simulink model "Proyecto_R2018a"  (R2018a)
settings: Solver=VariableStepAuto  StartTime=0.0  StopTime=3
undefined symbols (not defined in the file): alfa_inicial, area_mem, c, cte_kp, d, delta_f, fs, k, m, perm, Q, r1, r_ambiente1, r_ambiente2, rho, v_sonido, vel_caminata, ventana_fft, ventana_fft_analisis, zoh_freq
libraries: dspvision x10, dspmtrx3 x4, dspxfrm3 x3
settings Model: PacingRate=0.110000  Creator=tobip  LastModifiedBy=tobip
settings SolverCC: SolverResetMethod=Robust
settings DataIOCC: ReturnWorkspaceOutputs=on
settings DebuggingCC: UnconnectedInputMsg=none  UnconnectedOutputMsg=none  UnconnectedLineMsg=none
settings ModelReferenceCC: EnableRefExpFcnMdlSchedulingChecks=off
settings SFSimCC: SimUseLocalCustomCode=on
settings RTWCC: Description=Generic Real-Time Target  RTWUseLocalCustomCode=on

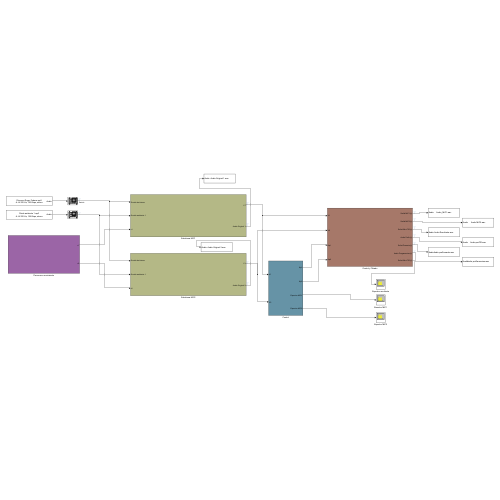
[thumbnail: Simulink's stored preview of the top-level diagram]
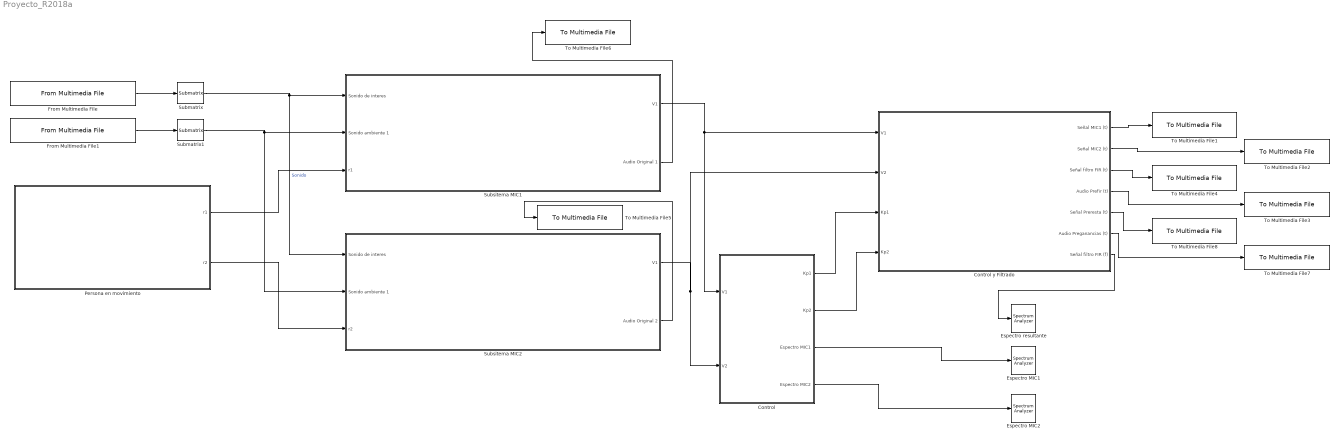
== system Proyecto_R2018a ==
  Control : Subsystem
  Control y Filtrado : Subsystem
  Espectro MIC1 : SpectrumAnalyzer  DefaultConfigurationName=spbscopes.SpectrumAnalyzerBlockCfg
  Espectro MIC2 : SpectrumAnalyzer  DefaultConfigurationName=spbscopes.SpectrumAnalyzerBlockCfg
  Espectro resultante : SpectrumAnalyzer  DefaultConfigurationName=spbscopes.SpectrumAnalyzerBlockCfg
  From Multimedia File : dspvision/From Multimedia File  inputFilename=C:\Users\tobip\Documents\Control\Proyecto final\Audios dato\Discurso Roger Federer.mp3  loop=on  numPlays=1  outputStreams=Audio only  videoDataType=single  audioDataType=double  inheritSampleTime=on  userDefinedSampleTime=1/30  noAudioOutput=off  isIntensityVideo=off  fourcc=RGB  colorVideoFormat=Separate color signals  outputEOF=off  dataOrg=Column-major  audioFrameSize=1  computeAudioFrameSize=off  outSamplingMode=Sample based
  From Multimedia File1 : dspvision/From Multimedia File  inputFilename=C:\Users\tobip\Documents\Control\Proyecto final\Audios dato\Ruido ambiente 1.mp3  loop=on  numPlays=1  outputStreams=Audio only  videoDataType=single  audioDataType=double  inheritSampleTime=on  userDefinedSampleTime=1/30  noAudioOutput=off  isIntensityVideo=off  fourcc=RGB  colorVideoFormat=Separate color signals  outputEOF=off  dataOrg=Column-major  audioFrameSize=1  computeAudioFrameSize=off  outSamplingMode=Sample based
  Persona en movimiento : Subsystem
  Submatrix : dspmtrx3/Submatrix  RowSpan=All rows  RowStartMode=First  RowStartIndex=1  RowEndMode=Middle  RowEndIndex=1  ColSpan=One column  ColStartMode=First  ColStartIndex=1  ColEndMode=Last  ColEndIndex=1
  Submatrix1 : dspmtrx3/Submatrix  RowSpan=All rows  RowStartMode=First  RowStartIndex=1  RowEndMode=Last  RowEndIndex=1  ColSpan=One column  ColStartMode=First  ColStartIndex=1  ColEndMode=Last  ColEndIndex=1
  Subsitema MIC1 : Subsystem
  Subsitema MIC2 : Subsystem
  To Multimedia File1 : dspvision/To Multimedia File  outputFilename=C:\Users\tobip\Documents\Control\Proyecto final\Audio_MIC1.wav  streamSelection=Audio only  videoCompressor=None (uncompressed)  audioCompressor=None (uncompressed)  imagePorts=Separate color signals  fileType=WAV  audioDatatype=16-bit integer  fourcc=RGB  videoQuality=75  mj2000CompFactor=10
  To Multimedia File2 : dspvision/To Multimedia File  outputFilename=C:\Users\tobip\Documents\Control\Proyecto final\Audio MIC2.wav  streamSelection=Audio only  videoCompressor=None (uncompressed)  audioCompressor=None (uncompressed)  imagePorts=Separate color signals  fileType=WAV  audioDatatype=16-bit integer  fourcc=RGB  videoQuality=75  mj2000CompFactor=10
  To Multimedia File3 : dspvision/To Multimedia File  outputFilename=C:\Users\tobip\Documents\Control\Proyecto final\Audio preFIR.wav  streamSelection=Audio only  videoCompressor=None (uncompressed)  audioCompressor=None (uncompressed)  imagePorts=Separate color signals  fileType=WAV  audioDatatype=16-bit integer  fourcc=RGB  videoQuality=75  mj2000CompFactor=10
  To Multimedia File4 : dspvision/To Multimedia File  outputFilename=C:\Users\tobip\Documents\Control\Proyecto final\Audio Resultante.wav  streamSelection=Audio only  videoCompressor=None (uncompressed)  audioCompressor=None (uncompressed)  imagePorts=Separate color signals  fileType=WAV  audioDatatype=16-bit integer  fourcc=RGB  videoQuality=75  mj2000CompFactor=10
  To Multimedia File5 : dspvision/To Multimedia File  outputFilename=C:\Users\tobip\Documents\Control\Proyecto final\Audio Original 2.wav  streamSelection=Audio only  videoCompressor=None (uncompressed)  audioCompressor=None (uncompressed)  imagePorts=Separate color signals  fileType=WAV  audioDatatype=16-bit integer  fourcc=RGB  videoQuality=75  mj2000CompFactor=10
  To Multimedia File6 : dspvision/To Multimedia File  outputFilename=C:\Users\tobip\Documents\Control\Proyecto final\Audio Original 1.wav  streamSelection=Audio only  videoCompressor=None (uncompressed)  audioCompressor=None (uncompressed)  imagePorts=Separate color signals  fileType=WAV  audioDatatype=16-bit integer  fourcc=RGB  videoQuality=75  mj2000CompFactor=10
  To Multimedia File7 : dspvision/To Multimedia File  outputFilename=C:\Users\tobip\Documents\Control\Proyecto final\Audio preGanancias.wav  streamSelection=Audio only  videoCompressor=None (uncompressed)  audioCompressor=None (uncompressed)  imagePorts=Separate color signals  fileType=WAV  audioDatatype=16-bit integer  fourcc=RGB  videoQuality=75  mj2000CompFactor=10
  To Multimedia File8 : dspvision/To Multimedia File  outputFilename=C:\Users\tobip\Documents\Control\Proyecto final\Audio preSumador.wav  streamSelection=Audio only  videoCompressor=None (uncompressed)  audioCompressor=None (uncompressed)  imagePorts=Separate color signals  fileType=WAV  audioDatatype=16-bit integer  fourcc=RGB  videoQuality=75  mj2000CompFactor=10
  wires:
  From Multimedia File/1 -> Submatrix/1
  From Multimedia File1/1 -> Submatrix1/1
  Submatrix/1 -> Subsitema MIC1/1(Sonido de interes), Subsitema MIC2/1(Sonido de interes)  "Sonido"
  Persona en movimiento/1(r1) -> Subsitema MIC1/3(r1)
  Control y Filtrado/1(Señal MIC1 (t)) -> To Multimedia File1/1
  Control y Filtrado/2(Señal MIC2 (t)) -> To Multimedia File2/1
  Control y Filtrado/3(Señal filtro FIR (t)) -> To Multimedia File4/1
  Control y Filtrado/4(Audio Prefir (t)) -> To Multimedia File3/1
  Control y Filtrado/7(Señal filtro FIR (f)) -> Espectro resultante/1
  Submatrix1/1 -> Subsitema MIC1/2(Sonido ambiente 1), Subsitema MIC2/2(Sonido ambiente 1)
  Persona en movimiento/2(r2) -> Subsitema MIC2/3(r2)
  Subsitema MIC1/2(Audio Original 1) -> To Multimedia File6/1
  Subsitema MIC2/2(Audio Original 2) -> To Multimedia File5/1
  Subsitema MIC1/1(V1) -> Control y Filtrado/1(V1), Control/1(V1)
  Subsitema MIC2/1(V1) -> Control y Filtrado/2(V2), Control/2(V2)
  Control/1(Kp1) -> Control y Filtrado/3(Kp1)
  Control/2(Kp2) -> Control y Filtrado/4(Kp2)
  Control/3(Espectro MIC1) -> Espectro MIC1/1
  Control/4(Espectro MIC2) -> Espectro MIC2/1
  Control y Filtrado/5(Señal Preresta (t)) -> To Multimedia File8/1
  Control y Filtrado/6(Audio Preganancias (t)) -> To Multimedia File7/1

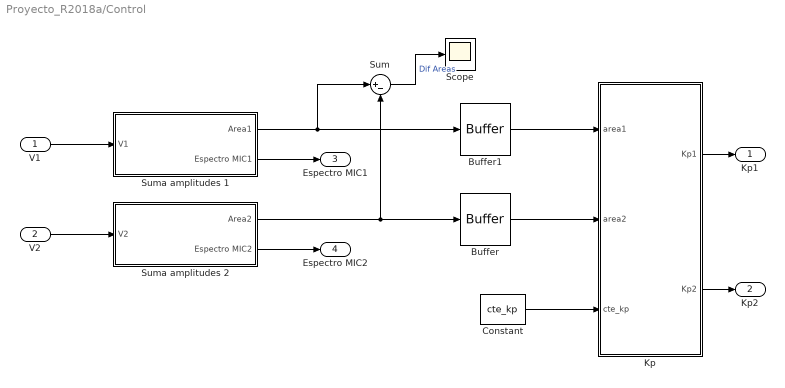
== system Proyecto_R2018a/Control ==
  V1 : Inport
  V2 : Inport  Port=2
  Buffer : Buffer  N=10  V=9  OutputFrames=off
  Buffer1 : Buffer  N=10  V=9  OutputFrames=off
  Constant : Constant  Value=cte_kp
  Kp : MATLAB Function  TreatAsAtomicUnit=on
  Scope : Scope
  Sum : Sum  Inputs=|+-
  Suma amplitudes 1 : Subsystem
  Suma amplitudes 2 : Subsystem
  Kp1 : Outport
  Kp2 : Outport  Port=2
  Espectro MIC1 : Outport  Port=3
  Espectro MIC2 : Outport  Port=4
  wires:
  Kp/1(Kp1) -> Kp1/1
  Constant/1 -> Kp/3(cte_kp)
  V1/1 -> Suma amplitudes 1/1(V1)
  V2/1 -> Suma amplitudes 2/1(V2)
  Kp/2(Kp2) -> Kp2/1
  Suma amplitudes 1/2(Espectro MIC1) -> Espectro MIC1/1
  Suma amplitudes 2/2(Espectro MIC2) -> Espectro MIC2/1
  Sum/1 -> Scope/1  "Dif Areas"
  Suma amplitudes 1/1(Area1) -> Buffer1/1, Sum/1
  Suma amplitudes 2/1(Area2) -> Sum/2, Buffer/1
  Buffer/1 -> Kp/2(area2)
  Buffer1/1 -> Kp/1(area1)

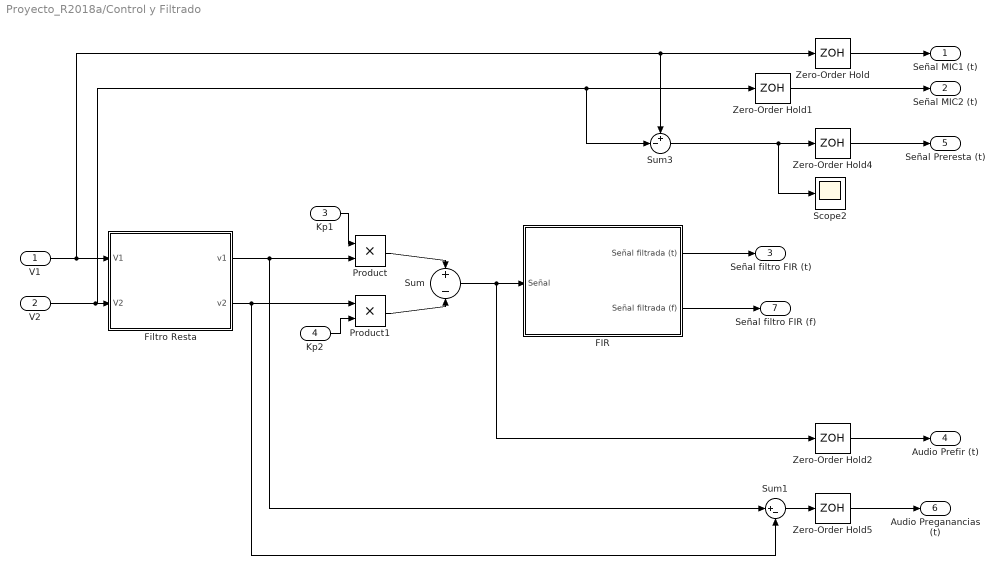
== system Proyecto_R2018a/Control y Filtrado ==
  V1 : Inport
  V2 : Inport  Port=2
  Kp1 : Inport  Port=3
  Kp2 : Inport  Port=4
  FIR : Subsystem
  Filtro Resta : MATLAB Function  TreatAsAtomicUnit=on
  Product : Product
  Product1 : Product
  Scope2 : Scope
  Sum : Sum  Inputs=+-
  Sum1 : Sum  Inputs=|+-
  Sum3 : Sum  Inputs=+-|
  Zero-Order Hold{,1..2,5} (4 alike) : ZeroOrderHold  SampleTime=1/fs
  Zero-Order Hold4 : ZeroOrderHold  SampleTime=1/44100
  Señal MIC1 (t) : Outport
  Señal MIC2 (t) : Outport  Port=2
  Señal filtro FIR (t) : Outport  Port=3
  Audio Prefir (t) : Outport  Port=4
  Señal Preresta (t) : Outport  Port=5
  Audio Preganancias (t) : Outport  Port=6
  Señal filtro FIR (f) : Outport  Port=7
  wires:
  V2/1 -> Filtro Resta/2(V2), Sum3/2, Zero-Order Hold1/1
  V1/1 -> Sum3/1, Zero-Order Hold/1, Filtro Resta/1(V1)
  Sum/1 -> FIR/1(Señal), Zero-Order Hold2/1
  FIR/2(Señal filtrada (f)) -> Señal filtro FIR (f)/1
  FIR/1(Señal filtrada (t)) -> Señal filtro FIR (t)/1
  Filtro Resta/2(v2) -> Product1/1, Sum1/2
  Filtro Resta/1(v1) -> Product/2, Sum1/1
  Zero-Order Hold/1 -> Señal MIC1 (t)/1
  Zero-Order Hold1/1 -> Señal MIC2 (t)/1
  Zero-Order Hold2/1 -> Audio Prefir (t)/1
  Sum1/1 -> Zero-Order Hold5/1
  Product1/1 -> Sum/2
  Product/1 -> Sum/1
  Sum3/1 -> Zero-Order Hold4/1, Scope2/1
  Kp1/1 -> Product/1
  Kp2/1 -> Product1/2
  Zero-Order Hold4/1 -> Señal Preresta (t)/1
  Zero-Order Hold5/1 -> Audio Preganancias (t)/1

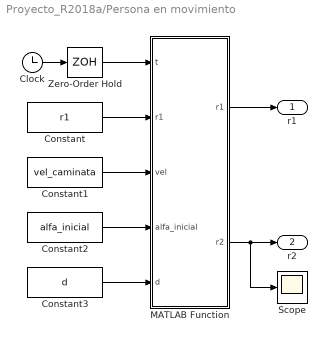
== system Proyecto_R2018a/Persona en movimiento ==
  Clock : Clock
  Constant : Constant  Value=r1
  Constant1 : Constant  Value=vel_caminata
  Constant2 : Constant  Value=alfa_inicial
  Constant3 : Constant  Value=d
  MATLAB Function : MATLAB Function  TreatAsAtomicUnit=on
  Scope : Scope
  Zero-Order Hold : ZeroOrderHold  SampleTime=0.1
  r1 : Outport
  r2 : Outport  Port=2
  wires:
  Constant/1 -> MATLAB Function/2("r1 ")
  Constant3/1 -> MATLAB Function/5(d)
  Constant2/1 -> MATLAB Function/4(alfa_inicial)
  Constant1/1 -> MATLAB Function/3(vel)
  Clock/1 -> Zero-Order Hold/1
  MATLAB Function/1(r1) -> r1/1
  Zero-Order Hold/1 -> MATLAB Function/1(t)
  MATLAB Function/2(r2) -> r2/1, Scope/1

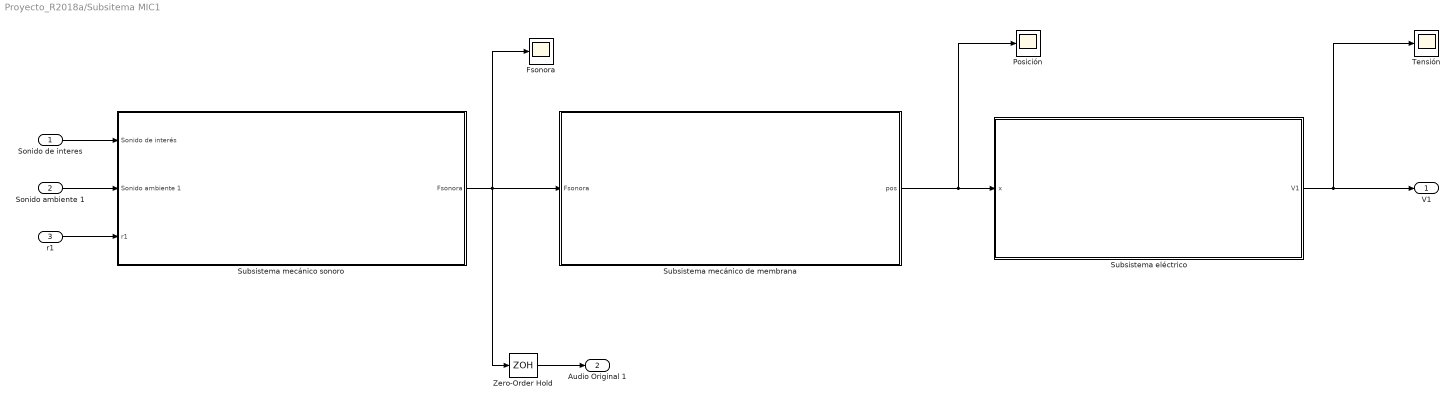
== system Proyecto_R2018a/Subsitema MIC1 ==
  Sonido de interes : Inport
  Sonido ambiente 1 : Inport  Port=2
  r1 : Inport  Port=3
  Fsonora : Scope
  Posición : Scope
  Subsistema eléctrico : Subsystem
  Subsistema mecánico de membrana : Subsystem
  Subsistema mecánico sonoro : Subsystem
  Tensión : Scope
  Zero-Order Hold : ZeroOrderHold  SampleTime=1/fs
  V1 : Outport
  Audio Original 1 : Outport  Port=2
  wires:
  Subsistema mecánico de membrana/1(pos) -> Posición/1, Subsistema eléctrico/1(x)
  Sonido de interes/1 -> Subsistema mecánico sonoro/1(Sonido de interés)
  Subsistema eléctrico/1(V1) -> Tensión/1, V1/1
  Subsistema mecánico sonoro/1(Fsonora) -> Fsonora/1, Zero-Order Hold/1, Subsistema mecánico de membrana/1(Fsonora)
  Sonido ambiente 1/1 -> Subsistema mecánico sonoro/2(Sonido ambiente 1)
  r1/1 -> Subsistema mecánico sonoro/3(r1)
  Zero-Order Hold/1 -> Audio Original 1/1

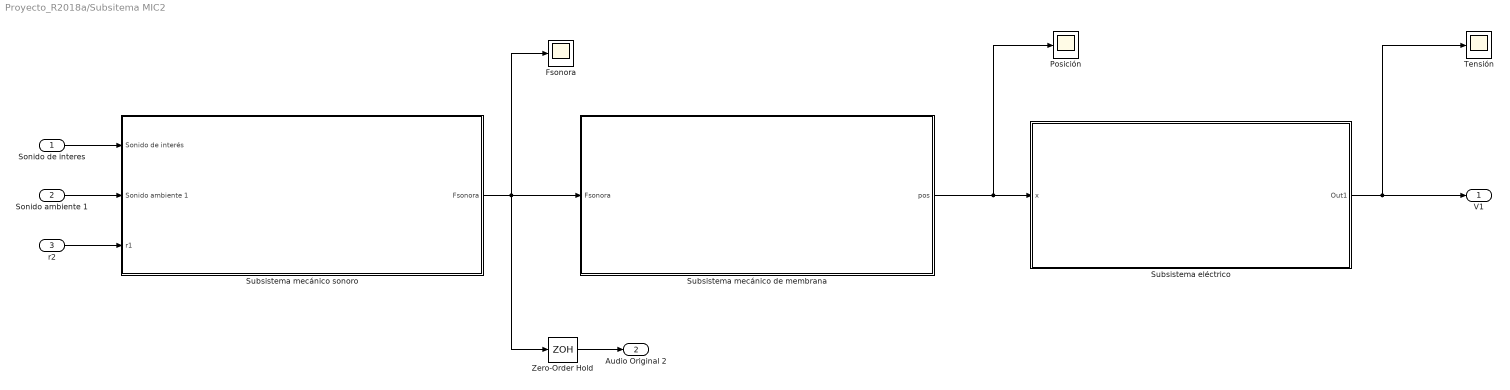
== system Proyecto_R2018a/Subsitema MIC2 ==
  Sonido de interes : Inport
  Sonido ambiente 1 : Inport  Port=2
  r2 : Inport  Port=3
  Fsonora : Scope
  Posición : Scope
  Subsistema eléctrico : Subsystem
  Subsistema mecánico de membrana : Subsystem
  Subsistema mecánico sonoro : Subsystem
  Tensión : Scope
  Zero-Order Hold : ZeroOrderHold  SampleTime=1/fs
  V1 : Outport
  Audio Original 2 : Outport  Port=2
  wires:
  Subsistema mecánico de membrana/1(pos) -> Posición/1, Subsistema eléctrico/1(x)
  Sonido de interes/1 -> Subsistema mecánico sonoro/1(Sonido de interés)
  Subsistema eléctrico/1(Out1) -> Tensión/1, V1/1
  Subsistema mecánico sonoro/1(Fsonora) -> Zero-Order Hold/1, Fsonora/1, Subsistema mecánico de membrana/1(Fsonora)
  Sonido ambiente 1/1 -> Subsistema mecánico sonoro/2(Sonido ambiente 1)
  r2/1 -> Subsistema mecánico sonoro/3(r1)
  Zero-Order Hold/1 -> Audio Original 2/1

== system Proyecto_R2018a/Control/Suma amplitudes 1 ==
  V1 : Inport
  Constant : Constant  Value=delta_f
  FFT : Subsystem
  MATLAB Function : MATLAB Function  TreatAsAtomicUnit=on
  Sum of Elements : Sum  Inputs=+
  Area1 : Outport
  Espectro MIC1 : Outport  Port=2
  wires:
  FFT/1(A) -> MATLAB Function/1(A)
  Constant/1 -> MATLAB Function/2(delta_f)
  MATLAB Function/1(areas) -> Sum of Elements/1
  Sum of Elements/1 -> Area1/1
  V1/1 -> FFT/1(In1)
  FFT/2(MIC1) -> Espectro MIC1/1

== system Proyecto_R2018a/Control/Suma amplitudes 2 ==
  V2 : Inport
  Constant : Constant  Value=delta_f
  MATLAB Function : MATLAB Function  TreatAsAtomicUnit=on
  Subsystem : Subsystem
  Sum of Elements : Sum  Inputs=+
  Area2 : Outport
  Espectro MIC2 : Outport  Port=2
  wires:
  Subsystem/1(A) -> MATLAB Function/1(A)
  Constant/1 -> MATLAB Function/2(delta_f)
  MATLAB Function/1(areas) -> Sum of Elements/1
  Sum of Elements/1 -> Area2/1
  V2/1 -> Subsystem/1(In1)
  Subsystem/2(MIC2) -> Espectro MIC2/1

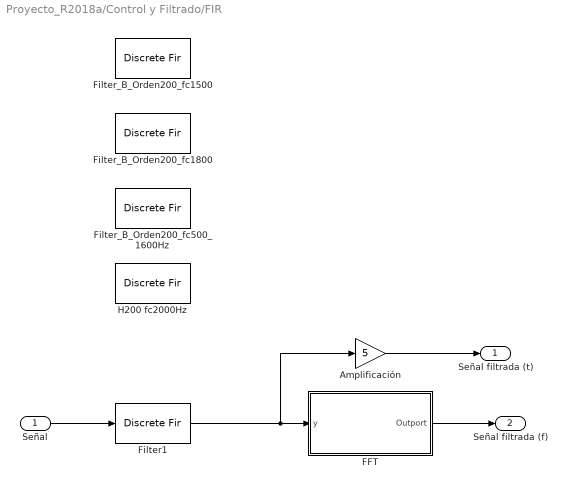
== system Proyecto_R2018a/Control y Filtrado/FIR ==
  Señal : Inport
  Amplificación : Gain  Gain=5
  FFT : Subsystem
  Filter1 : DiscreteFir  Tag=BlockMethodSubSystem  Coefficients=[0 -2.46968087486229999e-06 -3.07570330301983584e-05 -0.000118398297516965302 -0.000298367075036484037 -0.000596227803309950849 -0.00102003077952711506 -0.00154756625881359144 -0.00211289076768585247 -0.00259518747306043901 -0.00281365562212182018 -0.00253195194747434741 -0.00147460264563965674 0.00064414461322387991 0.00408104805501018075 0.00901875177176652762 0.0155214581908035953 0.0234991010213631106 0.0326874432853242192 0.0426497872392069197 0.0528029801451961808 0.0624665952648715134 0.070930220073032374 0.0775304241645051739 0.0817268652809263335 0.0831665725577227094 0.0817268652809263335 0.0775304241645051739 0.070930220073032374 0.0624665952648715134 0.0528029801451961808 0.0426497872392069197 0.0326874432853242192 0.0234991010213631106 0.0155214581908035953 0.00901875177176652762 0.00408104805501018075 0.00064414461322387991 -0.00147460264563965674 -0.00253195194747434741 -0.00281365562212182018 -0.00259518747306043901 -0.00211289076768585247 -0.00154756625881359144 -0.00102003077952711506 -0.000596227803309950849 -0.000298367075036484037 -0.000118398297516965302 -3.07570330301983584e-05 -2.46968087486229999e-06 0]
  Filter_B_Orden200_fc1500 : DiscreteFir  Tag=BlockMethodSubSystem  Coefficients=[0 2.11514125222930549e-07 1.00093934765138096e-06 2.50662436979156886e-06 4.71763254290821587e-06 7.45535130819729324e-06 1.03710140877794857e-05 1.2960590087806268e-05 1.45973519410186672e-05 1.45811762675124996e-05 1.22023273134778345e-05 6.81618827244323951e-06 -2.07578339154207704e-06 -1.47446077930910027e-05 -3.11583144423782112e-05 -5.09193211148811369e-05 -7.32215020803920553e-05 -9.68332887952996719e-05 -0.000120112140303127817 -0.000141054205202763115 -0.000157381003729514476 -0.000166662556647139825 -0.000166473685437744368 -0.00015457735079446705 -0.000129126060727848284 -8.88697665733315106e-05 -3.33564884044779432e-05 3.68896166032006936e-05 0.000120228712346331866 0.000213819912830098396 0.000313604278663653989 0.000414367756397579403 0.000509891865637218319 0.000593195126311718709 0.000656862556488219465 0.000693454334739479331 0.000695978258336398588 0.000658404344862743309 0.000576194261678405215 0.000446813676266662413 0.000270192532359212259 4.90970521410024542e-05 -0.000210621758123884174 -0.000499934975730347594 -0.000806724111547534105 -0.00111606896143020282 -0.00141074282481386303 -0.00167191115831235291 -0.00188001685492420584 -0.00201582207294112928 -0.00206156366447221876 -0.00200216760345560841 -0.00182645822084354721 -0.0015282913035907222 -0.00110753688360242983 -0.000570838357529814943 6.79202371766113587e-05 0.00078749732174142491 0.00155957185340557065 0.00234944320823486348 0.00311715878165994996 0.00381905210809447421 0.00440965014053728861 0.00484388441406833313 0.00507951851693627058 0.00507968498761981503 0.0048154097481520608 0.00426799261879337762 0.00343110924951585535 0.00231250356255708039 0.000935150787564285099 -0.000662210741248886155 -0.00242525619795645655 -0.00428500615435206331 -0.00615952594606015199 -0.00795636728195464604 -0.00957568849089815606 -0.0109139524588171416 -0.0118680670103581479 -0.0123398031736713185 -0.0122403041952631221 -0.0114944838213977812 -0.0100451073342442999 -0.0078563537756842685 -0.00491667285846230425 -0.00124077487520772665 0.00312937443093690539 0.0081246409678302229 0.0136499315738288548 0.019586515496723484 0.0257953968596963713 0.0321216271410308465 0.0383994009130048802 0.0444577386408763556 0.0501265293153456901 0.0552426847697761667 0.0596561479180048454 0.0632354994835633705 0.065872922121823177 0.067488306600615014 0.0680323207557864684 0.067488306600615014 0.065872922121823177 0.0632354994835633705 0.0596561479180048454 0.0552426847697761667 0.0501265293153456901 0.0444577386408763556 0.0383994009130048802 0.0321216271410308465 0.0257953968596963713 0.019586515496723484 0.0136499315738288548 0.0081246409678302229 0.00312937443093690539 -0.00124077487520772665 -0.00491667285846230425 -0.0078563537756842685 -0.0100451073342442999 -0.0114944838213977812 -0.0122403041952631221 -0.0123398031736713185 -0.0118680670103581479 -0.0109139524588171416 -0.00957568849089815606 -0.00795636728195464604 -0.00615952594606015199 -0.00428500615435206331 -0.00242525619795645655 -0.000662210741248886155 0.000935150787564285099 0.00231250356255708039 0.00343110924951585535 0.00426799261879337762 0.0048154097481520608 0.00507968498761981503 0.00507951851693627058 0.00484388441406833313 0.00440965014053728861 0.00381905210809447421 0.00311715878165994996 0.00234944320823486348 0.00155957185340557065 0.00078749732174142491 6.79202371766113587e-05 -0.000570838357529814943 -0.00110753688360242983 -0.0015282913035907222 -0.00182645822084354721 -0.00200216760345560841 -0.00206156366447221876 -0.00201582207294112928 -0.00188001685492420584 -0.00167191115831235291 -0.00141074282481386303 -0.00111606896143020282 -0.000806724111547534105 -0.000499934975730347594 -0.000210621758123884174 4.90970521410024542e-05 0.000270192532359212259 0.000446813676266662413 0.000576194261678405215 0.000658404344862743309 0.000695978258336398588 0.000693454334739479331 0.000656862556488219465 0.000593195126311718709 0.000509891865637218319 0.000414367756397579403 0.000313604278663653989 ...(+711 chars)]
  Filter_B_Orden200_fc1800 : DiscreteFir  Tag=BlockMethodSubSystem  Coefficients=[0 2.11514125222930549e-07 1.00093934765138096e-06 2.50662436979156886e-06 4.71763254290821587e-06 7.45535130819729324e-06 1.03710140877794857e-05 1.2960590087806268e-05 1.45973519410186672e-05 1.45811762675124996e-05 1.22023273134778345e-05 6.81618827244323951e-06 -2.07578339154207704e-06 -1.47446077930910027e-05 -3.11583144423782112e-05 -5.09193211148811369e-05 -7.32215020803920553e-05 -9.68332887952996719e-05 -0.000120112140303127817 -0.000141054205202763115 -0.000157381003729514476 -0.000166662556647139825 -0.000166473685437744368 -0.00015457735079446705 -0.000129126060727848284 -8.88697665733315106e-05 -3.33564884044779432e-05 3.68896166032006936e-05 0.000120228712346331866 0.000213819912830098396 0.000313604278663653989 0.000414367756397579403 0.000509891865637218319 0.000593195126311718709 0.000656862556488219465 0.000693454334739479331 0.000695978258336398588 0.000658404344862743309 0.000576194261678405215 0.000446813676266662413 0.000270192532359212259 4.90970521410024542e-05 -0.000210621758123884174 -0.000499934975730347594 -0.000806724111547534105 -0.00111606896143020282 -0.00141074282481386303 -0.00167191115831235291 -0.00188001685492420584 -0.00201582207294112928 -0.00206156366447221876 -0.00200216760345560841 -0.00182645822084354721 -0.0015282913035907222 -0.00110753688360242983 -0.000570838357529814943 6.79202371766113587e-05 0.00078749732174142491 0.00155957185340557065 0.00234944320823486348 0.00311715878165994996 0.00381905210809447421 0.00440965014053728861 0.00484388441406833313 0.00507951851693627058 0.00507968498761981503 0.0048154097481520608 0.00426799261879337762 0.00343110924951585535 0.00231250356255708039 0.000935150787564285099 -0.000662210741248886155 -0.00242525619795645655 -0.00428500615435206331 -0.00615952594606015199 -0.00795636728195464604 -0.00957568849089815606 -0.0109139524588171416 -0.0118680670103581479 -0.0123398031736713185 -0.0122403041952631221 -0.0114944838213977812 -0.0100451073342442999 -0.0078563537756842685 -0.00491667285846230425 -0.00124077487520772665 0.00312937443093690539 0.0081246409678302229 0.0136499315738288548 0.019586515496723484 0.0257953968596963713 0.0321216271410308465 0.0383994009130048802 0.0444577386408763556 0.0501265293153456901 0.0552426847697761667 0.0596561479180048454 0.0632354994835633705 0.065872922121823177 0.067488306600615014 0.0680323207557864684 0.067488306600615014 0.065872922121823177 0.0632354994835633705 0.0596561479180048454 0.0552426847697761667 0.0501265293153456901 0.0444577386408763556 0.0383994009130048802 0.0321216271410308465 0.0257953968596963713 0.019586515496723484 0.0136499315738288548 0.0081246409678302229 0.00312937443093690539 -0.00124077487520772665 -0.00491667285846230425 -0.0078563537756842685 -0.0100451073342442999 -0.0114944838213977812 -0.0122403041952631221 -0.0123398031736713185 -0.0118680670103581479 -0.0109139524588171416 -0.00957568849089815606 -0.00795636728195464604 -0.00615952594606015199 -0.00428500615435206331 -0.00242525619795645655 -0.000662210741248886155 0.000935150787564285099 0.00231250356255708039 0.00343110924951585535 0.00426799261879337762 0.0048154097481520608 0.00507968498761981503 0.00507951851693627058 0.00484388441406833313 0.00440965014053728861 0.00381905210809447421 0.00311715878165994996 0.00234944320823486348 0.00155957185340557065 0.00078749732174142491 6.79202371766113587e-05 -0.000570838357529814943 -0.00110753688360242983 -0.0015282913035907222 -0.00182645822084354721 -0.00200216760345560841 -0.00206156366447221876 -0.00201582207294112928 -0.00188001685492420584 -0.00167191115831235291 -0.00141074282481386303 -0.00111606896143020282 -0.000806724111547534105 -0.000499934975730347594 -0.000210621758123884174 4.90970521410024542e-05 0.000270192532359212259 0.000446813676266662413 0.000576194261678405215 0.000658404344862743309 0.000695978258336398588 0.000693454334739479331 0.000656862556488219465 0.000593195126311718709 0.000509891865637218319 0.000414367756397579403 0.000313604278663653989 ...(+711 chars)]
  Filter_B_Orden200_fc500_1600Hz : DiscreteFir  Tag=BlockMethodSubSystem  Coefficients=[0 -3.55324752461809841e-07 -1.14041164662054229e-06 -1.86555151808696453e-06 -1.99844780883798536e-06 -1.03117503681064552e-06 1.45062710751347741e-06 5.70289528973608542e-06 1.17693159029814948e-05 1.94448656927964283e-05 2.82621895124256615e-05 3.75049240470417836e-05 4.62502611344708104e-05 5.34408510414543662e-05 5.79836863954314837e-05 5.88710269009623936e-05 5.53158980566520483e-05 4.68924195295184699e-05 3.36693962809190553e-05 1.63244395128763006e-05 -3.77444374118628878e-06 -2.453220038109486e-05 -4.31457047987660692e-05 -5.61862277492814434e-05 -5.97494327243870303e-05 -4.96722181784016028e-05 -2.18103772002809209e-05 2.76346086120937394e-05 0.000101756893313425151 0.000202578002872316965 0.000330695331954048983 0.000484976370934371733 0.000662328426985930993 0.000857572264827437562 0.00106344444062398498 0.00127074710823718118 0.0014686558861857909 0.00164518631562104219 0.00178780802395475213 0.0018841836077030836 0.0019229972643288473 0.00189482722409228983 0.00179300697511287107 0.00161441401740641485 0.0013601221987472544 0.00103585517795217862 0.000652184596068289225 0.000224427194425909913 -0.00022778983727046132 -0.000681307141145609443 -0.00111054518170260381 -0.00148891652354738281 -0.00179048116367318505 -0.00199176515444643909 -0.00207364314459349474 -0.0020231703767315209 -0.00183524054863001091 -0.00151394393656255908 -0.00107350608403622406 -0.000538701511402984025 5.53408815078556784e-05 0.000663994493666133687 0.00123467192903057438 0.00170902033542422215 0.00202571129447411602 0.00212371962214221886 0.00194594664007262993 0.00144301027073342526 0.000576999157387270015 -0.000675026961659274034 -0.00231801155623287836 -0.00433656156585883468 -0.00669348216553504807 -0.00932933927728997296 -0.0121631565101997467 -0.0150942974724516503 -0.0180055222248230451 -0.0207671413150356775 -0.0232421259844599291 -0.0252919725618051955 -0.0267830664686852619 -0.0275932500724108756 -0.027618271722570361 -0.0267777828722388159 -0.0250205575078153546 -0.0223286335031159487 -0.0187201182440967645 -0.014250459181509658 -0.00901205114390197723 -0.00313213274256277877 0.00323099015437159709 0.00989326969472957042 0.0166515838433948446 0.0232914672367314154 0.0295955653449251239 0.0353524284672399047 0.0403652375807131078 0.04446005042715033 0.0474931739498184249 0.0493573075805954289 0.0499861590665064068 0.0493573075805954289 0.0474931739498184249 0.04446005042715033 0.0403652375807131078 0.0353524284672399047 0.0295955653449251239 0.0232914672367314154 0.0166515838433948446 0.00989326969472957042 0.00323099015437159709 -0.00313213274256277877 -0.00901205114390197723 -0.014250459181509658 -0.0187201182440967645 -0.0223286335031159487 -0.0250205575078153546 -0.0267777828722388159 -0.027618271722570361 -0.0275932500724108756 -0.0267830664686852619 -0.0252919725618051955 -0.0232421259844599291 -0.0207671413150356775 -0.0180055222248230451 -0.0150942974724516503 -0.0121631565101997467 -0.00932933927728997296 -0.00669348216553504807 -0.00433656156585883468 -0.00231801155623287836 -0.000675026961659274034 0.000576999157387270015 0.00144301027073342526 0.00194594664007262993 0.00212371962214221886 0.00202571129447411602 0.00170902033542422215 0.00123467192903057438 0.000663994493666133687 5.53408815078556784e-05 -0.000538701511402984025 -0.00107350608403622406 -0.00151394393656255908 -0.00183524054863001091 -0.0020231703767315209 -0.00207364314459349474 -0.00199176515444643909 -0.00179048116367318505 -0.00148891652354738281 -0.00111054518170260381 -0.000681307141145609443 -0.00022778983727046132 0.000224427194425909913 0.000652184596068289225 0.00103585517795217862 0.0013601221987472544 0.00161441401740641485 0.00179300697511287107 0.00189482722409228983 0.0019229972643288473 0.0018841836077030836 0.00178780802395475213 0.00164518631562104219 0.0014686558861857909 0.00127074710823718118 0.00106344444062398498 0.000857572264827437562 0.000662328426985930993 0.000484976370934371733 0.000330695331954048983 ...(+708 chars)]
  H200 fc2000Hz : DiscreteFir  Tag=BlockMethodSubSystem  Coefficients=[-5.56928887965323996e-05 1.65011438245537004e-05 8.97404129389855278e-05 0.000159235323802665862 0.00022009162972417537 0.000267507778546905491 0.000297028076662561244 0.00030485366062257119 0.000288200030555739591 0.000245675511305965986 0.000177641669329940406 8.6506699720296273e-05 -2.31018469780051173e-05 -0.00014433637834937926 -0.000268342086729793134 -0.000384707364236210015 -0.00048215215755155206 -0.000549426670478966937 -0.000576363543252263362 -0.000554999408859523633 -0.000480660081578202522 -0.000352890851136748013 -0.000176112058154881163 4.01080891230722538e-05 0.0002812463338075579 0.000528528322799664608 0.000760142225443803492 0.000952907949042803453 0.00108429460403765884 0.00113463045342545839 0.00108931159601457291 0.00094079311035012215 0.000690143237104743116 0.000347959694228160642 -6.55123016736293336e-05 -0.000521160190085571311 -0.000982705755809358409 -0.00140926525119598289 -0.00175861601479996091 -0.001990934889977244 -0.00207270564165747606 -0.00198044699745618087 -0.00170389625705465349 -0.00124829972377997456 -0.000635511796707235511 9.63124522686815125e-05 0.000894536087431914602 0.00169534580071897009 0.0024283810074139326 0.00302238837764083959 0.00341148451645994577 0.00354151851327269909 0.00337597368177574393 0.00290084170646281786 0.00212794664955293479 0.00109629064041346963 -0.000128867164522033134 -0.00145931071589772685 -0.00278945929549263881 -0.00400395802404863912 -0.00498677619654774081 -0.00563115432140427145 -0.00584961657959357211 -0.00558319945973669973 -0.00480904907338582793 -0.00354561337216146395 -0.00185479953038198927 0.000159326606607727535 0.00235546635562724864 0.00456352016844470149 0.00659611134894932602 0.00826250699229939302 0.00938400051612865889 0.00980963996366138874 0.00943108496947073389 0.0081953652910344444 0.00611440066924413047 0.00327032343009041803 -0.000184088132840851902 -0.00403022302427255476 -0.00799367568943868192 -0.0117590911319403208 -0.0149890162285861283 -0.0173456171069947714 -0.0185138545635019809 -0.0182245363907261523 -0.0162756038401307805 -0.0125500678039269838 -0.00702918815483403927 0.000200222721545358193 0.0089451122912353586 0.0189124119976689584 0.029721990975099373 0.0409256801261550299 0.052031266702432348 0.0625299886144426165 0.0719257851026266215 0.079764407724826486 0.0856604757140051049 0.0893206756611368557 0.0905615500562179931 0.0893206756611368557 0.0856604757140051049 0.079764407724826486 0.0719257851026266215 0.0625299886144426165 0.052031266702432348 0.0409256801261550299 0.029721990975099373 0.0189124119976689584 0.0089451122912353586 0.000200222721545358193 -0.00702918815483403927 -0.0125500678039269838 -0.0162756038401307805 -0.0182245363907261523 -0.0185138545635019809 -0.0173456171069947714 -0.0149890162285861283 -0.0117590911319403208 -0.00799367568943868192 -0.00403022302427255476 -0.000184088132840851902 0.00327032343009041803 0.00611440066924413047 0.0081953652910344444 0.00943108496947073389 0.00980963996366138874 0.00938400051612865889 0.00826250699229939302 0.00659611134894932602 0.00456352016844470149 0.00235546635562724864 0.000159326606607727535 -0.00185479953038198927 -0.00354561337216146395 -0.00480904907338582793 -0.00558319945973669973 -0.00584961657959357211 -0.00563115432140427145 -0.00498677619654774081 -0.00400395802404863912 -0.00278945929549263881 -0.00145931071589772685 -0.000128867164522033134 0.00109629064041346963 0.00212794664955293479 0.00290084170646281786 0.00337597368177574393 0.00354151851327269909 0.00341148451645994577 0.00302238837764083959 0.0024283810074139326 0.00169534580071897009 0.000894536087431914602 9.63124522686815125e-05 -0.000635511796707235511 -0.00124829972377997456 -0.00170389625705465349 -0.00198044699745618087 -0.00207270564165747606 -0.001990934889977244 -0.00175861601479996091 -0.00140926525119598289 -0.000982705755809358409 -0.000521160190085571311 -6.55123016736293336e-05 0.000347959694228160642 0.000690143237104743116 0.00094079311035012215 ...(+746 chars)]
  Señal filtrada (t) : Outport
  Señal filtrada (f) : Outport  Port=2
  wires:
  FFT/1(Outport) -> Señal filtrada (f)/1
  Amplificación/1 -> Señal filtrada (t)/1
  Señal/1 -> Filter1/1
  Filter1/1 -> Amplificación/1, FFT/1(y)

== system Proyecto_R2018a/Subsitema MIC1/Subsistema eléctrico ==
  x : Inport
  Constant : Constant  Value=area_mem*perm
  Constant1 : Constant  Value=Q
  Divide : Product  Inputs=*/
  Divide1 : Product  Inputs=*/
  V1 : Outport
  wires:
  x/1 -> Divide/2
  Constant/1 -> Divide/1
  Divide/1 -> Divide1/2  "Capacitancia"
  Divide1/1 -> V1/1
  Constant1/1 -> Divide1/1

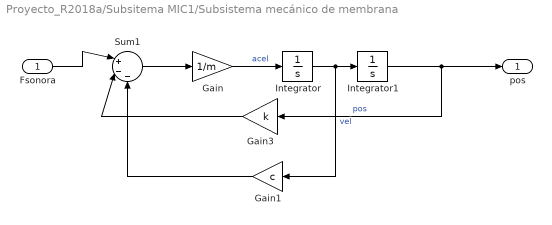
== system Proyecto_R2018a/Subsitema MIC1/Subsistema mecánico de membrana ==
  Fsonora : Inport
  Gain : Gain  Gain=1/m
  Gain1 : Gain  Gain=c
  Gain3 : Gain  Gain=k
  Integrator : Integrator
  Integrator1 : Integrator
  Sum1 : Sum  Inputs=|+--
  pos : Outport
  wires:
  Integrator1/1 -> Gain3/1, pos/1  "pos"
  Integrator/1 -> Gain1/1, Integrator1/1  "vel"
  Fsonora/1 -> Sum1/1
  Gain3/1 -> Sum1/2
  Sum1/1 -> Gain/1
  Gain/1 -> Integrator/1  "acel"
  Gain1/1 -> Sum1/3

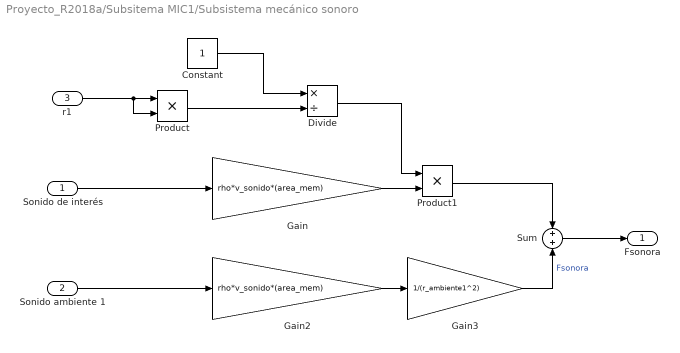
== system Proyecto_R2018a/Subsitema MIC1/Subsistema mecánico sonoro ==
  Sonido de interés : Inport
  Sonido ambiente 1 : Inport  Port=2
  r1 : Inport  Port=3
  Constant : Constant
  Divide : Product  Inputs=*/
  Gain : Gain  Gain=rho*v_sonido*(area_mem)
  Gain2 : Gain  Gain=rho*v_sonido*(area_mem)
  Gain3 : Gain  Gain=1/(r_ambiente1^2)
  Product : Product
  Product1 : Product
  Sum : Sum
  Fsonora : Outport
  wires:
  Gain/1 -> Product1/2
  Sonido de interés/1 -> Gain/1
  Gain2/1 -> Gain3/1
  Gain3/1 -> Sum/2  "Fsonora"
  Sonido ambiente 1/1 -> Gain2/1
  Sum/1 -> Fsonora/1
  r1/1 -> Product/2, Product/1
  Product/1 -> Divide/2
  Constant/1 -> Divide/1
  Divide/1 -> Product1/1
  Product1/1 -> Sum/1

== system Proyecto_R2018a/Subsitema MIC2/Subsistema eléctrico ==
  x : Inport
  Constant : Constant  Value=area_mem*perm
  Constant1 : Constant  Value=Q
  Divide : Product  Inputs=*/
  Divide1 : Product  Inputs=*/
  Out1 : Outport
  wires:
  x/1 -> Divide/2
  Constant/1 -> Divide/1
  Divide/1 -> Divide1/2  "Capacitancia"
  Divide1/1 -> Out1/1
  Constant1/1 -> Divide1/1

== system Proyecto_R2018a/Subsitema MIC2/Subsistema mecánico de membrana ==
  Fsonora : Inport
  Gain : Gain  Gain=1/m
  Gain1 : Gain  Gain=c
  Gain3 : Gain  Gain=k
  Integrator : Integrator
  Integrator1 : Integrator
  Sum1 : Sum  Inputs=|+--
  pos : Outport
  wires:
  Integrator1/1 -> Gain3/1, pos/1  "pos"
  Integrator/1 -> Gain1/1, Integrator1/1  "vel"
  Fsonora/1 -> Sum1/1
  Gain3/1 -> Sum1/2
  Sum1/1 -> Gain/1
  Gain/1 -> Integrator/1  "acel"
  Gain1/1 -> Sum1/3

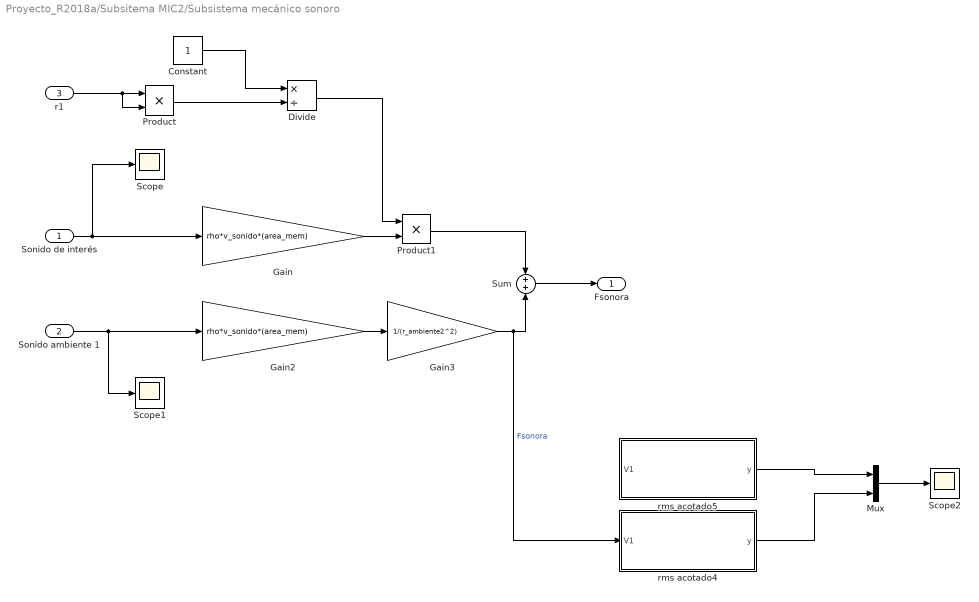
== system Proyecto_R2018a/Subsitema MIC2/Subsistema mecánico sonoro ==
  Sonido de interés : Inport
  Sonido ambiente 1 : Inport  Port=2
  r1 : Inport  Port=3
  Constant : Constant
  Divide : Product  Inputs=*/
  Gain : Gain  Gain=rho*v_sonido*(area_mem)
  Gain2 : Gain  Gain=rho*v_sonido*(area_mem)
  Gain3 : Gain  Gain=1/(r_ambiente2^2)
  Mux : Mux  Inputs=2
  Product : Product
  Product1 : Product
  Scope : Scope
  Scope1 : Scope
  Scope2 : Scope
  Sum : Sum
  rms acotado4 : Subsystem
  rms acotado5 : Subsystem
  Fsonora : Outport
  wires:
  Gain/1 -> Product1/2
  Sonido de interés/1 -> Gain/1, Scope/1
  Gain2/1 -> Gain3/1
  Gain3/1 -> rms acotado4/1(V1), Sum/2  "Fsonora"
  Sonido ambiente 1/1 -> Scope1/1, Gain2/1
  Sum/1 -> Fsonora/1
  rms acotado5/1(y) -> Mux/1
  rms acotado4/1(y) -> Mux/2
  Mux/1 -> Scope2/1
  r1/1 -> Product/2, Product/1
  Product/1 -> Divide/2
  Constant/1 -> Divide/1
  Divide/1 -> Product1/1
  Product1/1 -> Sum/1

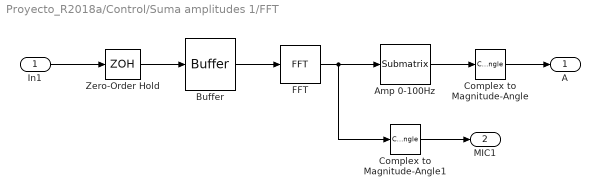
== system Proyecto_R2018a/Control/Suma amplitudes 1/FFT ==
  In1 : Inport
  Amp 0-100Hz : dspmtrx3/Submatrix  RowSpan=Range of rows  RowStartMode=Index  RowStartIndex=1  RowEndMode=Index  RowEndIndex=30  ColSpan=One column  ColStartMode=First  ColStartIndex=1  ColEndMode=Last  ColEndIndex=1
  Buffer : Buffer  N=ventana_fft  V=ventana_fft_analisis-1  OutputFrames=off
  Complex to Magnitude-Angle : ComplexToMagnitudeAngle  Output=Magnitude
  Complex to Magnitude-Angle1 : ComplexToMagnitudeAngle  Output=Magnitude
  FFT : dspxfrm3/FFT  FFTImplementation=Auto  CompMethod=Table lookup  TableOpt=NEW  TableOptActive=Speed  BitRevOrder=off  Normalize=off  InheritFFTLength=on  FFTLength=64  WrapInput=on  roundingMode=Floor  overflowMode=off  firstCoeffDataTypeStr=Inherit: Same word length as input  firstCoeffLastDataTypeStr=Inherit: Same word length as input  outputMin=[]  outputMax=[]
  Zero-Order Hold : ZeroOrderHold  SampleTime=zoh_freq
  A : Outport
  MIC1 : Outport  Port=2
  wires:
  Complex to Magnitude-Angle/1 -> A/1
  FFT/1 -> Complex to Magnitude-Angle1/1, Amp 0-100Hz/1
  In1/1 -> Zero-Order Hold/1
  Buffer/1 -> FFT/1
  Zero-Order Hold/1 -> Buffer/1
  Amp 0-100Hz/1 -> Complex to Magnitude-Angle/1
  Complex to Magnitude-Angle1/1 -> MIC1/1

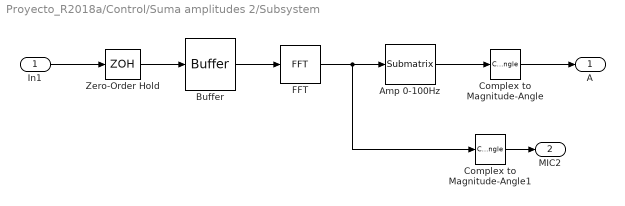
== system Proyecto_R2018a/Control/Suma amplitudes 2/Subsystem ==
  In1 : Inport
  Amp 0-100Hz : dspmtrx3/Submatrix  RowSpan=Range of rows  RowStartMode=Index  RowStartIndex=1  RowEndMode=Index  RowEndIndex=30  ColSpan=One column  ColStartMode=First  ColStartIndex=1  ColEndMode=Last  ColEndIndex=1
  Buffer : Buffer  N=ventana_fft  V=ventana_fft_analisis-1  OutputFrames=off
  Complex to Magnitude-Angle : ComplexToMagnitudeAngle  Output=Magnitude
  Complex to Magnitude-Angle1 : ComplexToMagnitudeAngle  Output=Magnitude
  FFT : dspxfrm3/FFT  FFTImplementation=Auto  CompMethod=Table lookup  TableOpt=NEW  TableOptActive=Speed  BitRevOrder=off  Normalize=off  InheritFFTLength=on  FFTLength=64  WrapInput=on  roundingMode=Floor  overflowMode=off  firstCoeffDataTypeStr=Inherit: Same word length as input  firstCoeffLastDataTypeStr=Inherit: Same word length as input  outputMin=[]  outputMax=[]
  Zero-Order Hold : ZeroOrderHold  SampleTime=zoh_freq
  A : Outport
  MIC2 : Outport  Port=2
  wires:
  In1/1 -> Zero-Order Hold/1
  Complex to Magnitude-Angle/1 -> A/1
  FFT/1 -> Complex to Magnitude-Angle1/1, Amp 0-100Hz/1
  Buffer/1 -> FFT/1
  Zero-Order Hold/1 -> Buffer/1
  Amp 0-100Hz/1 -> Complex to Magnitude-Angle/1
  Complex to Magnitude-Angle1/1 -> MIC2/1

== system Proyecto_R2018a/Control y Filtrado/FIR/FFT ==
  y : Inport
  Buffer : Buffer  N=4410  OutputFrames=off
  Complex to Magnitude-Angle : ComplexToMagnitudeAngle  Output=Magnitude
  FFT : dspxfrm3/FFT  FFTImplementation=Auto  CompMethod=Table lookup  TableOpt=NEW  TableOptActive=Speed  BitRevOrder=off  Normalize=off  InheritFFTLength=on  FFTLength=64  WrapInput=on  roundingMode=Floor  overflowMode=off  firstCoeffDataTypeStr=Inherit: Same word length as input  firstCoeffLastDataTypeStr=Inherit: Same word length as input  outputMin=[]  outputMax=[]
  Zero-Order Hold : ZeroOrderHold  SampleTime=zoh_freq
  Outport : Outport
  wires:
  Buffer/1 -> FFT/1
  Complex to Magnitude-Angle/1 -> Outport/1
  y/1 -> Zero-Order Hold/1
  Zero-Order Hold/1 -> Buffer/1
  FFT/1 -> Complex to Magnitude-Angle/1

== system Proyecto_R2018a/Subsitema MIC2/Subsistema mecánico sonoro/rms acotado4 ==
  V1 : Inport
  Buffer : Buffer  N=20  OutputFrames=off
  MATLAB Function : MATLAB Function  TreatAsAtomicUnit=on
  Zero-Order Hold : ZeroOrderHold  SampleTime=zoh_freq
  y : Outport
  wires:
  MATLAB Function/1(y) -> y/1
  Buffer/1 -> MATLAB Function/1(u)
  V1/1 -> Zero-Order Hold/1
  Zero-Order Hold/1 -> Buffer/1

== system Proyecto_R2018a/Subsitema MIC2/Subsistema mecánico sonoro/rms acotado5 ==
  V1 : Inport
  Buffer : Buffer  N=20  OutputFrames=off
  MATLAB Function : MATLAB Function  TreatAsAtomicUnit=on
  Zero-Order Hold : ZeroOrderHold  SampleTime=zoh_freq
  y : Outport
  wires:
  MATLAB Function/1(y) -> y/1
  Buffer/1 -> MATLAB Function/1(u)
  V1/1 -> Zero-Order Hold/1
  Zero-Order Hold/1 -> Buffer/1

== matlab function Proyecto_R2018a/Control y Filtrado/Filtro Resta ==
  data: V1 input; V2 input; v1 output; v2 output
function [v1,v2]= fcn(V1,V2)

%% ========= Logica 1 =============
dif_amp = 0.00005;
    % if abs(V1-V2) <= dif_amp
    %     v1 = V1;
    %     v2 = V2;
    % elseif ((abs(V1-V2) > dif_amp) && (V1 > 0) && (V2 > 0) && (V1>V2))
    %     v1 = V1 - V2;
    %     v2 = V2;
    % elseif ((abs(V1-V2) > dif_amp) && (V1 > 0) && (V2 > 0) && (V2>V1))
    %     v2 = V2 - V1;
    %     v1 = V1;
    % elseif ((abs(V1-V2) > dif_amp) && (V1 < 0) && (V2 > 0) && (abs(V1)>abs(V2)))
    %     v1 = V1 + V2;
    %     v2 = V2;
    % elseif ((abs(V1-V2) > dif_amp) && (V1 < 0) && (V2 > 0) && (abs(V1)<abs(V2)))
    %     v2 = V1 + V2;
    %     v1 = V1;
    % elseif ((abs(V1-V2) > dif_amp) && (V1 > 0) && (V2 < 0) && (abs(V1)<abs(V2)))
    %     v2 = V1 + V2;
    %     v1 = V1;
    % elseif ((abs(V1-V2) > dif_amp) && (V1 > 0) && (V2 < 0) && (abs(V1)>abs(V2)))
    %     v1 = V1 + V2;
    %     v2 = V2;
    % else
    %     v1 = 0;
    %     v2 = 0;
    % end

%% ========= Logica 2 ===========
 % if abs(V1-V2) <= dif_amp
 %        v1 = V1;
 %        v2 = V2;
 %    else
 %        v1 = V1 - V2;
 %        v2 = V2 - V1;
 %    end
%% ========== Logica 3 ==========
%Lógica teniendo en cuenta la diferencias de áreas que se obtiene al
%calcular ganancias (No resultó)

%% ========== Logica 4 ==========
% v1 = V1; %No se realiza ninguna operación
% v2 = V2;

%% ========== Logica 5 ==========
if abs(V1-V2) <= dif_amp
        v1 = V1;
        v2 = V2;
else
    v1 = V1 - V2;
    v2 = V2 - V1;
end
end

== matlab function Proyecto_R2018a/Subsitema MIC2/Subsistema mecánico sonoro/rms acotado4/MATLAB Function ==
  data: u input; y output
function y = fcn(u)
% y=0;
%     for i=1:length(u)
%         y = y + u(i)^2;
%     end
%     y=sqrt(y);
    y = sqrt(mean(u.^2));

== matlab function Proyecto_R2018a/Persona en movimiento/MATLAB Function ==
  settings: updateMethod=DISCRETE
  data: t input; r1 output; r1 input; vel input; alfa_inicial input; d input; r2 output
function [r1, r2] = fcn(t, r1, vel, alfa_inicial, d)

persistent h fig

omega = vel/r1;
alfa = alfa_inicial + omega*t;
r2 = sqrt((r1^2) + (d^2) - 2*r1*d*cos(alfa));   %Distancia a mic2

x1 = r1*cos(alfa);
y1 = r1*sin(alfa);

% Inicializar el gráfico
if isempty(h)
    fig = figure('Name', 'Caminata en el plano', 'NumberTitle', 'off');
    h = plot(0, 0, 'ro', 'MarkerSize', 10, 'MarkerFaceColor', 'r');
    axis([-1 1 -1 1]); % Ajusta los límites según el rango de tu simulación
    grid on;
    xlabel('X (m)');
    ylabel('Y (m)');
    title('Caminata en el plano');
end

% Actualizar el punto
if ishandle(h)  % Cambiado de 'isvalid' a 'ishandle'
    set(h, 'XData', x1, 'YData', y1);
    hold on
     plot(d/2, 0, 'ro' ,'MarkerSize', 30, 'MarkerFaceColor', 'k');
    plot(0, 0, 'ro' ,'MarkerSize', 4, 'MarkerFaceColor', 'b');
    plot(d, 0, 'ro' ,'MarkerSize', 4, 'MarkerFaceColor', 'b');
    hold off
    drawnow;
end
end

== matlab function Proyecto_R2018a/Subsitema MIC2/Subsistema mecánico sonoro/rms acotado5/MATLAB Function ==
  data: u input; y output
function y = fcn(u)
% y=0;
%     for i=1:length(u)
%         y = y + u(i)^2;
%     end
%     y=sqrt(y);
    y = sqrt(mean(u.^2));

== matlab function Proyecto_R2018a/Control/Kp ==
  data: area1 input; area2 input; Kp1 output; cte_kp input; Kp2 output
function [Kp1,Kp2]= fcn(area1,area2,cte_kp)

%Las ganancias variaria de entre 0 y cte_kp

area_max = max(area1(end), area2(end));
delta_area = area1(end)-area2(end);
deltas_areas = area1-area2;


    if delta_area <= 0 && abs(delta_area) >= 50
        Kp1 = cte_kp - abs(delta_area)*(cte_kp/area_max);
        Kp2 = cte_kp + abs(delta_area)*(cte_kp/area_max);
    elseif delta_area > 0 && abs(delta_area) >= 50
        Kp1 = cte_kp + abs(delta_area)*(cte_kp/area_max);
        Kp2 = cte_kp - abs(delta_area)*(cte_kp/area_max);
    else
        Kp1 = cte_kp;
        Kp2 = cte_kp;
    end

    for i=1:1:length(deltas_areas)
        if abs(deltas_areas(i)) < 50
            Kp1 = cte_kp;
            Kp2 = cte_kp;
        end
    end

== matlab function Proyecto_R2018a/Control/Suma amplitudes 1/MATLAB Function ==
  data: A input; areas output; delta_f input
function areas = fcn(A, delta_f)

areas = A.* delta_f;

== matlab function Proyecto_R2018a/Control/Suma amplitudes 2/MATLAB Function ==
  data: A input; areas output; delta_f input
function areas = fcn(A, delta_f)

areas = A.* delta_f;
